simulink model "ShifterLogic"  (R2023a)
settings: Solver=FixedStepDiscrete  StartTime=0.0  StopTime=10.0  FixedStep=Ts  RelTol=1e-3
values from neighbouring files (symbols this model uses):
  AbsoluteMaxGear = 30    [Startup.m]
settings Model: Creator=Carlos  LastModifiedBy=Carlos
settings OptimizationCC: DefaultUnderspecifiedDataType=single  OptimizeBlockIOStorage=off  BufferReuse=off  ReuseModelBlockBuffer=off  GlobalBufferReuse=off  ExpressionFolding=off  EnableMemcpy=off  PassReuseOutputArgsAs=Individual arguments  LocalBlockOutputs=off  ZeroExternalMemoryAtStartup=off  ZeroInternalMemoryAtStartup=off  OptimizeDataStoreBuffers=off  BusAssignmentInplaceUpdate=off  OptimizationLevel=level0  OptimizationCustomize=off  EfficientTunableParamExpr=on
settings DebuggingCC: ParameterTunabilityLossMsg=error
settings HardwareCC: ProdBitPerInt=16  ProdBitPerPointer=16  ProdBitPerSizeT=16  ProdBitPerPtrDiffT=16  ProdLargestAtomicFloat=None  ProdWordSize=8  ProdHWDeviceType=Atmel->AVR
settings SFSimCC: MATLABDynamicMemAlloc=off  SimTargetLang=C++
settings RTWCC: Description=Embedded Coder  SystemTargetFile=ert.tlc  GenCodeOnly=on  TemplateMakefile=ert_default_tmf  TargetLang=C++
settings CodeAppCC: ForceParamTrailComments=on  IgnoreCustomStorageClasses=off  OperatorAnnotations=on  SimulinkDataObjDesc=on  SFDataObjDesc=on  InsertBlockDesc=on
settings ERTTargetCC: TargetLangStandard=C++11 (ISO)  GenerateSampleERTMain=on  CodeInterfacePackaging=C++ class  SupportNonFinite=off  SupportContinuousTime=on  RootIOFormat=Structure reference  ERTCustomFileTemplate=example_file_process.tlc

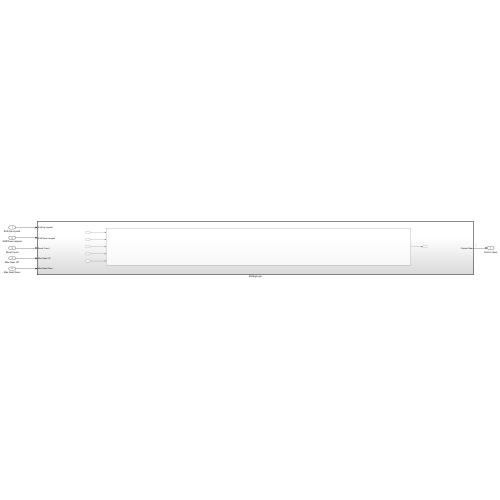
[thumbnail: Simulink's stored preview of the top-level diagram]
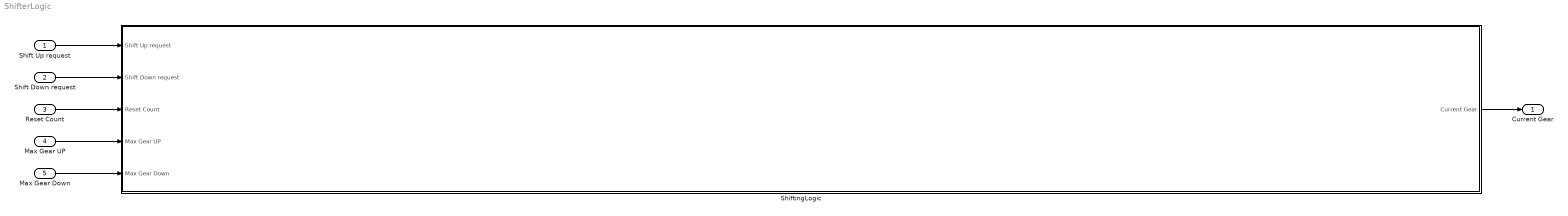
== system ShifterLogic ==
  Shift Up request : Inport  OutDataTypeStr=uint8
  Shift Down request : Inport  Port=2  OutDataTypeStr=uint8
  Reset Count : Inport  Port=3  OutDataTypeStr=uint8
  Max Gear UP : Inport  Port=4  OutDataTypeStr=uint8
  Max Gear Down : Inport  Port=5  OutDataTypeStr=uint8
  ShiftingLogic : Subsystem  TreatAsAtomicUnit=on
  Current Gear : Outport  OutDataTypeStr=int8
  wires:
  Shift Up request/1 -> ShiftingLogic/1(Shift Up request)
  Shift Down request/1 -> ShiftingLogic/2(Shift Down request)
  Reset Count/1 -> ShiftingLogic/3(Reset Count)
  Max Gear UP/1 -> ShiftingLogic/4(Max Gear UP)
  Max Gear Down/1 -> ShiftingLogic/5(Max Gear Down)
  ShiftingLogic/1(Current Gear) -> Current Gear/1

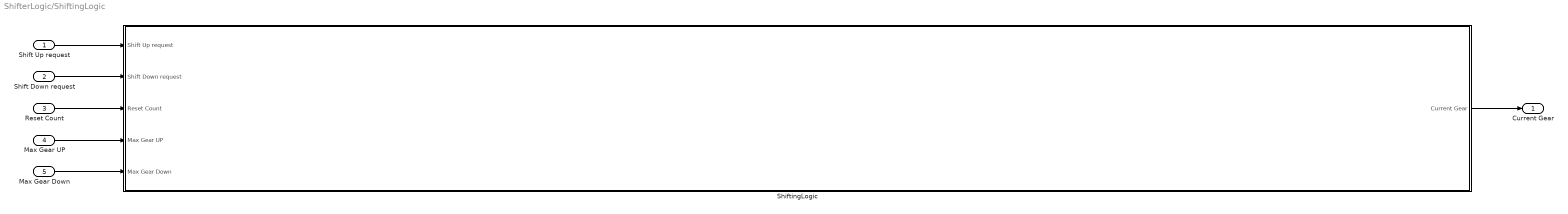
== system ShifterLogic/ShiftingLogic ==
  Shift Up request : Inport
  Shift Down request : Inport  Port=2
  Reset Count : Inport  Port=3
  Max Gear UP : Inport  Port=4
  Max Gear Down : Inport  Port=5
  ShiftingLogic : Subsystem  TreatAsAtomicUnit=on
  Current Gear : Outport
  wires:
  ShiftingLogic/1(Current Gear) -> Current Gear/1
  Max Gear UP/1 -> ShiftingLogic/4(Max Gear UP)
  Shift Up request/1 -> ShiftingLogic/1(Shift Up request)
  Shift Down request/1 -> ShiftingLogic/2(Shift Down request)
  Reset Count/1 -> ShiftingLogic/3(Reset Count)
  Max Gear Down/1 -> ShiftingLogic/5(Max Gear Down)

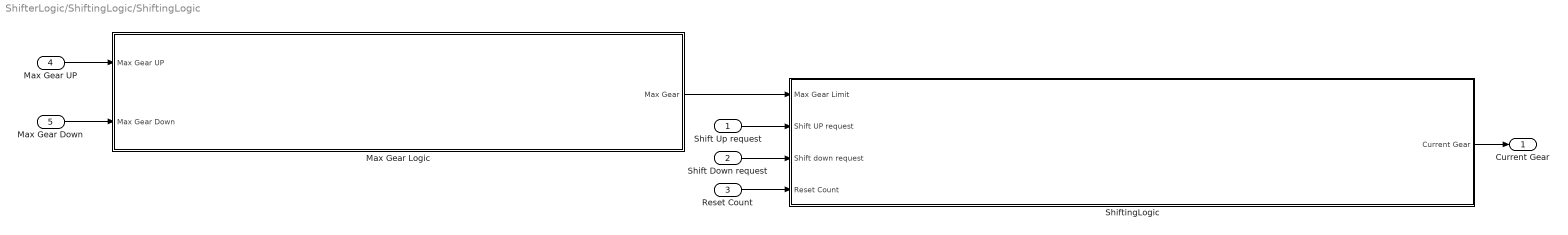
== system ShifterLogic/ShiftingLogic/ShiftingLogic ==
  Shift Up request : Inport  OutDataTypeStr=uint8
  Shift Down request : Inport  Port=2  OutDataTypeStr=uint8
  Reset Count : Inport  Port=3  OutDataTypeStr=uint8
  Max Gear UP : Inport  Port=4  OutDataTypeStr=uint8
  Max Gear Down : Inport  Port=5  OutDataTypeStr=uint8
  Max Gear Logic : Subsystem
  ShiftingLogic : Subsystem  TreatAsAtomicUnit=on
  Current Gear : Outport  OutDataTypeStr=int8
  wires:
  Shift Up request/1 -> ShiftingLogic/2(Shift UP request)
  Max Gear Logic/1(Max Gear) -> ShiftingLogic/1(Max Gear Limit)
  Max Gear UP/1 -> Max Gear Logic/1(Max Gear UP)
  ShiftingLogic/1(Current Gear) -> Current Gear/1
  Max Gear Down/1 -> Max Gear Logic/2(Max Gear Down)
  Reset Count/1 -> ShiftingLogic/4(Reset Count)
  Shift Down request/1 -> ShiftingLogic/3(Shift down request)

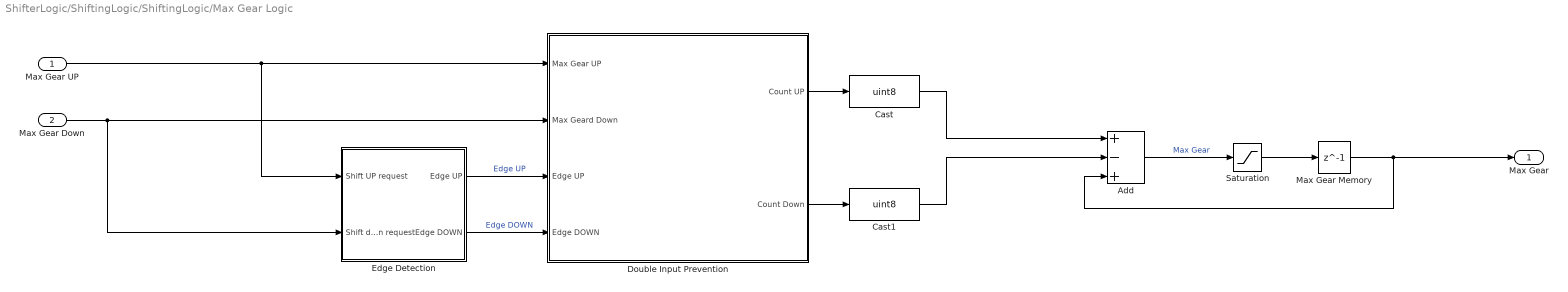
== system ShifterLogic/ShiftingLogic/ShiftingLogic/Max Gear Logic ==
  Max Gear UP : Inport
  Max Gear Down : Inport  Port=2
  Add : Sum  Inputs=+-+
  Cast : DataTypeConversion  OutDataTypeStr=uint8  SaturateOnIntegerOverflow=off  RndMeth=Floor
  Cast1 : DataTypeConversion  OutDataTypeStr=uint8  SaturateOnIntegerOverflow=off  RndMeth=Floor
  Double Input Prevention : Subsystem
  Edge Detection : Subsystem
  Max Gear Memory : Delay  DelayLength=1  InitialCondition=0
  Saturation : Saturate  UpperLimit=20  LowerLimit=1
  Max Gear : Outport
  wires:
  Max Gear Down/1 -> Double Input Prevention/2(Max Geard Down), Edge Detection/2(Shift down request)
  Double Input Prevention/1(Count UP) -> Cast/1
  Max Gear UP/1 -> Edge Detection/1(Shift UP request), Double Input Prevention/1(Max Gear UP)
  Double Input Prevention/2(Count Down) -> Cast1/1
  Edge Detection/2(Edge DOWN) -> Double Input Prevention/4(Edge DOWN)  "Edge DOWN"
  Max Gear Memory/1 -> Max Gear/1, Add/3
  Edge Detection/1(Edge UP) -> Double Input Prevention/3(Edge UP)  "Edge UP"
  Add/1 -> Saturation/1  "Max Gear"
  Saturation/1 -> Max Gear Memory/1
  Cast/1 -> Add/1
  Cast1/1 -> Add/2

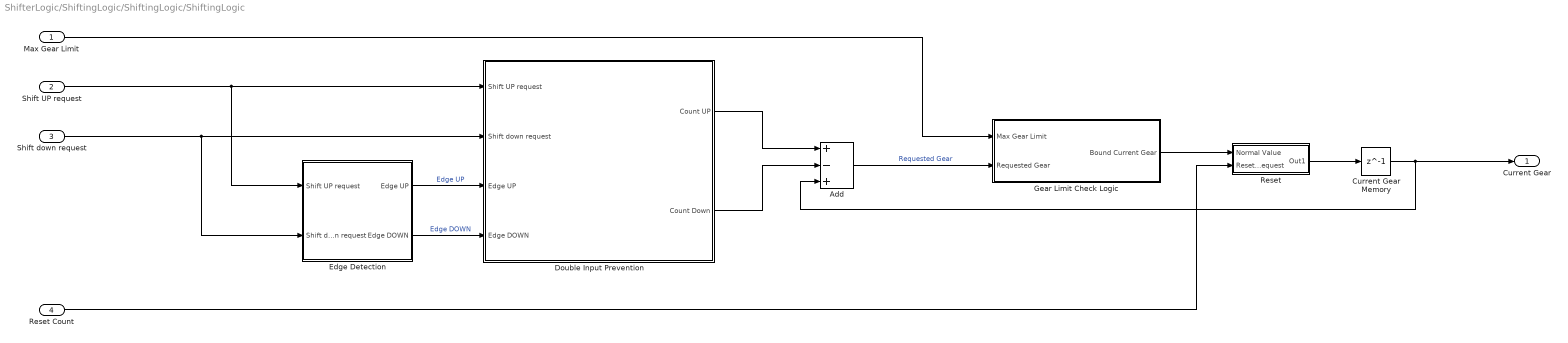
== system ShifterLogic/ShiftingLogic/ShiftingLogic/ShiftingLogic ==
  Max Gear Limit : Inport  OutDataTypeStr=uint8
  Shift UP request : Inport  Port=2  OutDataTypeStr=uint8
  Shift down request : Inport  Port=3  OutDataTypeStr=uint8
  Reset Count : Inport  Port=4  OutDataTypeStr=uint8
  Add : Sum  Inputs=+-+
  Current Gear Memory : Delay  DelayLength=1  InitialCondition=0
  Double Input Prevention : Subsystem
  Edge Detection : Subsystem
  Gear Limit Check Logic : Subsystem
  Reset : Subsystem
  Current Gear : Outport  OutDataTypeStr=int8
  wires:
  Current Gear Memory/1 -> Current Gear/1, Add/3
  Double Input Prevention/2(Count Down) -> Add/2
  Double Input Prevention/1(Count UP) -> Add/1
  Edge Detection/1(Edge UP) -> Double Input Prevention/3(Edge UP)  "Edge UP"
  Edge Detection/2(Edge DOWN) -> Double Input Prevention/4(Edge DOWN)  "Edge DOWN"
  Max Gear Limit/1 -> Gear Limit Check Logic/1(Max Gear Limit)
  Add/1 -> Gear Limit Check Logic/2(Requested Gear)  "Requested Gear"
  Shift down request/1 -> Edge Detection/2(Shift down request), Double Input Prevention/2(Shift down request)
  Shift UP request/1 -> Edge Detection/1(Shift UP request), Double Input Prevention/1(Shift UP request)
  Gear Limit Check Logic/1(Bound Current Gear) -> Reset/1(Normal Value)
  Reset Count/1 -> Reset/2(Reset Request)
  Reset/1(Out1) -> Current Gear Memory/1

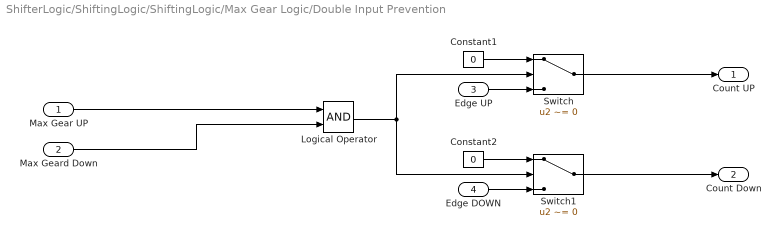
== system ShifterLogic/ShiftingLogic/ShiftingLogic/Max Gear Logic/Double Input Prevention ==
  Max Gear UP : Inport
  Max Geard Down : Inport  Port=2
  Edge UP : Inport  Port=3
  Edge DOWN : Inport  Port=4
  Constant1 : Constant  Value=0
  Constant2 : Constant  Value=0
  Logical Operator : Logic  AllPortsSameDT=off  OutDataTypeStr=boolean
  Switch : Switch  Criteria=u2 ~= 0  SaturateOnIntegerOverflow=off  InputSameDT=off
  Switch1 : Switch  Criteria=u2 ~= 0  SaturateOnIntegerOverflow=off  InputSameDT=off
  Count UP : Outport
  Count Down : Outport  Port=2
  wires:
  Switch/1 -> Count UP/1
  Constant1/1 -> Switch/1
  Logical Operator/1 -> Switch1/2, Switch/2
  Edge DOWN/1 -> Switch1/3
  Max Geard Down/1 -> Logical Operator/2
  Constant2/1 -> Switch1/1
  Max Gear UP/1 -> Logical Operator/1
  Switch1/1 -> Count Down/1
  Edge UP/1 -> Switch/3

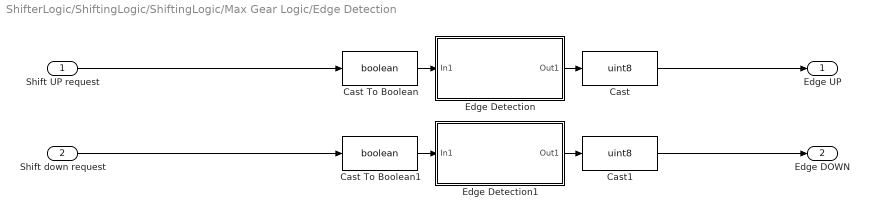
== system ShifterLogic/ShiftingLogic/ShiftingLogic/Max Gear Logic/Edge Detection ==
  Shift UP request : Inport
  Shift down request : Inport  Port=2
  Cast : DataTypeConversion  OutDataTypeStr=uint8  SaturateOnIntegerOverflow=off  RndMeth=Floor
  Cast To Boolean : DataTypeConversion  OutDataTypeStr=boolean  SaturateOnIntegerOverflow=off  RndMeth=Floor
  Cast To Boolean1 : DataTypeConversion  OutDataTypeStr=boolean  SaturateOnIntegerOverflow=off  RndMeth=Floor
  Cast1 : DataTypeConversion  OutDataTypeStr=uint8  SaturateOnIntegerOverflow=off  RndMeth=Floor
  Edge Detection : Subsystem
  Edge Detection1 : Subsystem
  Edge UP : Outport
  Edge DOWN : Outport  Port=2
  wires:
  Cast To Boolean1/1 -> Edge Detection1/1(In1)
  Edge Detection1/1(Out1) -> Cast1/1
  Edge Detection/1(Out1) -> Cast/1
  Cast To Boolean/1 -> Edge Detection/1(In1)
  Shift down request/1 -> Cast To Boolean1/1
  Cast/1 -> Edge UP/1
  Cast1/1 -> Edge DOWN/1
  Shift UP request/1 -> Cast To Boolean/1

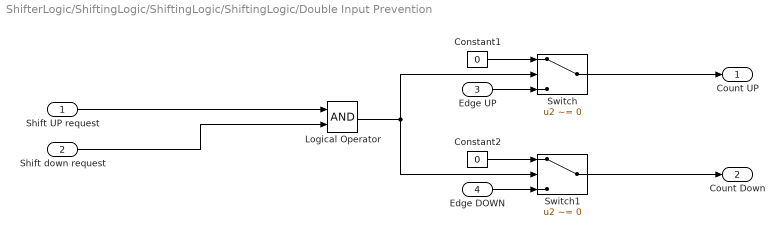
== system ShifterLogic/ShiftingLogic/ShiftingLogic/ShiftingLogic/Double Input Prevention ==
  Shift UP request : Inport
  Shift down request : Inport  Port=2
  Edge UP : Inport  Port=3
  Edge DOWN : Inport  Port=4
  Constant1 : Constant  Value=0
  Constant2 : Constant  Value=0
  Logical Operator : Logic  AllPortsSameDT=off  OutDataTypeStr=boolean
  Switch : Switch  Criteria=u2 ~= 0  SaturateOnIntegerOverflow=off  InputSameDT=off
  Switch1 : Switch  Criteria=u2 ~= 0  SaturateOnIntegerOverflow=off  InputSameDT=off
  Count UP : Outport
  Count Down : Outport  Port=2
  wires:
  Switch/1 -> Count UP/1
  Constant1/1 -> Switch/1
  Logical Operator/1 -> Switch1/2, Switch/2
  Edge DOWN/1 -> Switch1/3
  Shift down request/1 -> Logical Operator/2
  Constant2/1 -> Switch1/1
  Shift UP request/1 -> Logical Operator/1
  Switch1/1 -> Count Down/1
  Edge UP/1 -> Switch/3

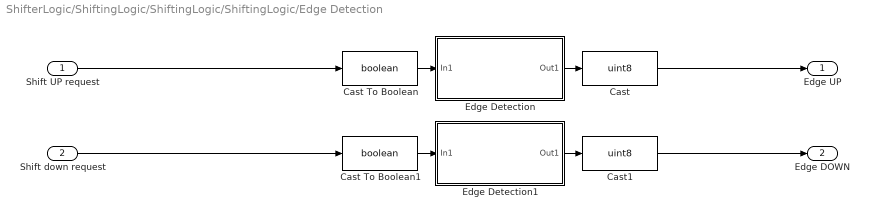
== system ShifterLogic/ShiftingLogic/ShiftingLogic/ShiftingLogic/Edge Detection ==
  Shift UP request : Inport
  Shift down request : Inport  Port=2
  Cast : DataTypeConversion  OutDataTypeStr=uint8  SaturateOnIntegerOverflow=off  RndMeth=Floor
  Cast To Boolean : DataTypeConversion  OutDataTypeStr=boolean  SaturateOnIntegerOverflow=off  RndMeth=Floor
  Cast To Boolean1 : DataTypeConversion  OutDataTypeStr=boolean  SaturateOnIntegerOverflow=off  RndMeth=Floor
  Cast1 : DataTypeConversion  OutDataTypeStr=uint8  SaturateOnIntegerOverflow=off  RndMeth=Floor
  Edge Detection : Subsystem
  Edge Detection1 : Subsystem
  Edge UP : Outport
  Edge DOWN : Outport  Port=2
  wires:
  Cast To Boolean1/1 -> Edge Detection1/1(In1)
  Edge Detection1/1(Out1) -> Cast1/1
  Edge Detection/1(Out1) -> Cast/1
  Cast To Boolean/1 -> Edge Detection/1(In1)
  Shift down request/1 -> Cast To Boolean1/1
  Cast/1 -> Edge UP/1
  Cast1/1 -> Edge DOWN/1
  Shift UP request/1 -> Cast To Boolean/1

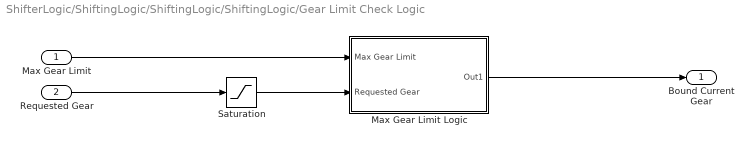
== system ShifterLogic/ShiftingLogic/ShiftingLogic/ShiftingLogic/Gear Limit Check Logic ==
  Max Gear Limit : Inport
  Requested Gear : Inport  Port=2
  Max Gear Limit Logic : Subsystem
  Saturation : Saturate  UpperLimit=AbsoluteMaxGear  LowerLimit=-1
  Bound Current Gear : Outport
  wires:
  Saturation/1 -> Max Gear Limit Logic/2(Requested Gear)
  Requested Gear/1 -> Saturation/1
  Max Gear Limit Logic/1(Out1) -> Bound Current Gear/1
  Max Gear Limit/1 -> Max Gear Limit Logic/1(Max Gear Limit)

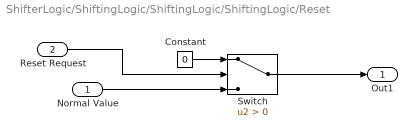
== system ShifterLogic/ShiftingLogic/ShiftingLogic/ShiftingLogic/Reset ==
  Normal Value : Inport
  Reset Request : Inport  Port=2
  Constant : Constant  Value=0
  Switch : Switch  Criteria=u2 > Threshold  SaturateOnIntegerOverflow=off  InputSameDT=off
  Out1 : Outport
  wires:
  Constant/1 -> Switch/1
  Switch/1 -> Out1/1
  Reset Request/1 -> Switch/2
  Normal Value/1 -> Switch/3

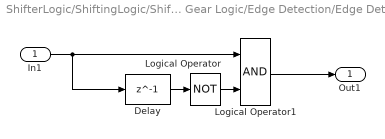
== system ShifterLogic/ShiftingLogic/ShiftingLogic/Max Gear Logic/Edge Detection/Edge Detection ==
  In1 : Inport
  Delay : Delay  DelayLength=1  InitialCondition=1  InputProcessing=Columns as channels (frame based)
  Logical Operator : Logic  Operator=NOT  Inputs=1
  Logical Operator1 : Logic
  Out1 : Outport
  wires:
  In1/1 -> Delay/1, Logical Operator1/1
  Logical Operator/1 -> Logical Operator1/2
  Delay/1 -> Logical Operator/1
  Logical Operator1/1 -> Out1/1

== system ShifterLogic/ShiftingLogic/ShiftingLogic/Max Gear Logic/Edge Detection/Edge Detection1 ==
  In1 : Inport
  Delay : Delay  DelayLength=1  InitialCondition=1  InputProcessing=Columns as channels (frame based)
  Logical Operator : Logic  Operator=NOT  Inputs=1
  Logical Operator1 : Logic
  Out1 : Outport
  wires:
  In1/1 -> Delay/1, Logical Operator1/1
  Logical Operator/1 -> Logical Operator1/2
  Delay/1 -> Logical Operator/1
  Logical Operator1/1 -> Out1/1

== system ShifterLogic/ShiftingLogic/ShiftingLogic/ShiftingLogic/Edge Detection/Edge Detection ==
  In1 : Inport
  Delay : Delay  DelayLength=1  InitialCondition=1  InputProcessing=Columns as channels (frame based)
  Logical Operator : Logic  Operator=NOT  Inputs=1
  Logical Operator1 : Logic
  Out1 : Outport
  wires:
  In1/1 -> Delay/1, Logical Operator1/1
  Logical Operator/1 -> Logical Operator1/2
  Delay/1 -> Logical Operator/1
  Logical Operator1/1 -> Out1/1

== system ShifterLogic/ShiftingLogic/ShiftingLogic/ShiftingLogic/Edge Detection/Edge Detection1 ==
  In1 : Inport
  Delay : Delay  DelayLength=1  InitialCondition=1  InputProcessing=Columns as channels (frame based)
  Logical Operator : Logic  Operator=NOT  Inputs=1
  Logical Operator1 : Logic
  Out1 : Outport
  wires:
  In1/1 -> Delay/1, Logical Operator1/1
  Logical Operator/1 -> Logical Operator1/2
  Delay/1 -> Logical Operator/1
  Logical Operator1/1 -> Out1/1

== system ShifterLogic/ShiftingLogic/ShiftingLogic/ShiftingLogic/Gear Limit Check Logic/Max Gear Limit Logic ==
  Max Gear Limit : Inport
  Requested Gear : Inport  Port=2
  Relational Operator : RelationalOperator  Operator=<  OutDataTypeStr=boolean  RndMeth=Simplest  InputSameDT=off
  Switch : Switch  Criteria=u2 ~= 0  SaturateOnIntegerOverflow=off  InputSameDT=off
  Out1 : Outport
  wires:
  Max Gear Limit/1 -> Switch/1, Relational Operator/1
  Requested Gear/1 -> Switch/3, Relational Operator/2
  Relational Operator/1 -> Switch/2
  Switch/1 -> Out1/1
